simulink model "sim20_8_3"  (R2017a)
settings: Solver=ode45  StartTime=0.0  StopTime=15  FixedStep=0.05  MaxStep=0.05  RelTol=1e-3
libraries: simulink x2
settings Model: Creator=asus  LastModifiedBy=Lenovo

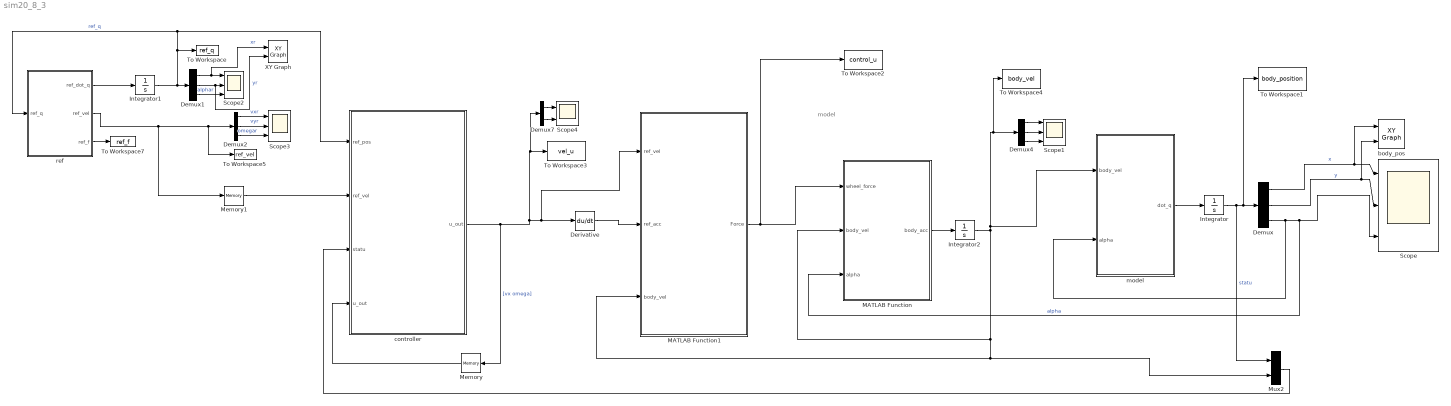
== system sim20_8_3 ==
  note: model
  Demux{,1..2,4} (4 alike) : Demux  Outputs=3
  Demux7 : Demux  Outputs=2
  Derivative : Derivative
  Integrator : Integrator  InitialCondition=[1; -1; pi/2;]  IgnoreLimit=on
  Integrator1 : Integrator  InitialCondition=[0;0;pi/4]
  Integrator2 : Integrator  InitialCondition=[0.2; 0; 0]
  MATLAB Function : MATLAB Function  TreatAsAtomicUnit=on
  MATLAB Function1 : MATLAB Function  TreatAsAtomicUnit=on
  Memory : Memory  X0=[0; 0]
  Memory1 : Memory  X0=[0.00001; 0.00001 ; 0.000001]
  Mux2 : Mux  Inputs=2
  Scope{,1..3} (4 alike) : Scope  NumInputPorts=3
  Scope4 : Scope  NumInputPorts=2
  To Workspace : ToWorkspace  VariableName=ref_q  SampleTime=-1
  To Workspace1 : ToWorkspace  VariableName=body_position  SampleTime=-1
  To Workspace2 : ToWorkspace  VariableName=control_u  SampleTime=-1
  To Workspace3 : ToWorkspace  VariableName=vel_u  SampleTime=-1
  To Workspace4 : ToWorkspace  VariableName=body_vel  SampleTime=-1
  To Workspace5 : ToWorkspace  VariableName=ref_vel  SampleTime=-1
  To Workspace7 : ToWorkspace  VariableName=ref_f  SampleTime=-1
  XY Graph : simulink/Sinks/XY Graph  xmin=-10  xmax=10  ymin=-10  ymax=10  st=-1
  body_pos : simulink/Sinks/XY Graph  xmin=-10  xmax=10  ymin=-10  ymax=10  st=-1
  controller : MATLAB Function  TreatAsAtomicUnit=on
  model : MATLAB Function  TreatAsAtomicUnit=on
  ref : MATLAB Function  TreatAsAtomicUnit=on
  wires:
  Demux2/2 -> Scope3/2  "vyr"
  Demux2/1 -> Scope3/1  "vxr"
  ref/2(ref_vel) -> Memory1/1, To Workspace5/1, Demux2/1
  Integrator/1 -> To Workspace1/1, Demux/1, Mux2/1  "statu"
  Demux1/3 -> Scope2/3  "alphar"
  Demux1/1 -> XY Graph/1, Scope2/1  "xr"
  Demux1/2 -> XY Graph/2, Scope2/2  "yr"
  Demux2/3 -> Scope3/3  "omegar"
  Demux/3 -> model/2(alpha), MATLAB Function/3(alpha), Scope/3  "alpha"
  Demux/1 -> body_pos/1, Scope/1  "x"
  Demux/2 -> body_pos/2, Scope/2  "y"
  ref/1(ref_dot_q) -> Integrator1/1
  Integrator1/1 -> ref/1(ref_q), controller/1(ref_pos), To Workspace/1, Demux1/1  "ref_q"
  Demux7/2 -> Scope4/2
  Demux7/1 -> Scope4/1
  model/1(dot_q) -> Integrator/1
  controller/1(u_out) -> MATLAB Function1/1(ref_vel), Derivative/1, Demux7/1, To Workspace3/1, Memory/1  "[vx omega]"
  Memory/1 -> controller/4("u_out ")
  Memory1/1 -> controller/2(ref_vel)
  ref/3(ref_f) -> To Workspace7/1
  Mux2/1 -> controller/3(statu)
  Integrator2/1 -> Mux2/2, MATLAB Function1/3(body_vel), MATLAB Function/2(body_vel), model/1(body_vel), To Workspace4/1, Demux4/1
  MATLAB Function/1(body_acc) -> Integrator2/1
  Demux4/1 -> Scope1/1
  Demux4/3 -> Scope1/3
  MATLAB Function1/1(Force) -> To Workspace2/1, MATLAB Function/1(wheel_force)
  Demux4/2 -> Scope1/2
  Derivative/1 -> MATLAB Function1/2(ref_acc)

== matlab function sim20_8_3/controller ==
  data: ref_pos input; ref_vel input; u_out output; statu input; u_out input
function u_out  = my_MPC_controller(ref_pos, ref_vel, statu, u_out)

% 程序上没有问题，在运动学模型上是可以完成任务的
% 最近修改时间：7.25 
% 基于运动学模型的MPC控制器
% u_out=[vx ;  omega]
% ref_vel=[xr yr alphar vr omegar]
% e = [ex ey ealpha]

Nc= 10; Np=20; %预测时域Np	控制时域Nc
T=0.05; 

% 测试是否能得到
%    statu=[2; -2; pi/2; 0.001; 0.001; 0.001];
%    u_out=[0; 0];
%    ref_pos=[0;0;pi/4]; ref_vel=[2; 0; 0];  
%% 底盘参数
d = 0.18;	l = 0.16;	m = 24;	Iz = 11.89;	c = 513.6; %轮胎侧偏刚度

%% 状态量                                                                           
x = statu(1);   y = statu(2);  alpha = statu(3); 
vx = statu(4);  vy = statu(5);    omega = statu(6);
                                      
                                                                            
xr=ref_pos(1);  yr=ref_pos(2);  alphar=ref_pos(3);
vxr=ref_vel(1); vyr=ref_vel(2); omegar=ref_vel(3);
                                                                                      
%控制量个数Nu
Nu=size(u_out,1);

%状态量个数Nx
statu_error=[x-xr;   y-yr;   alpha-alphar;]; 
Nx=size(statu_error,1);

% 控制矩阵求解(将连续矩阵转换为离散矩阵，采用近似算法  A=I+T*A(t),B=T*B(t))
% 此处：delta_X=AX+BU ————X=[a-r]=[X_I-Xr;Y_I-Yr;ALPHA_I-ALPHAr]statu_e=A*statu_e+B*u_e   %离散后的模型
    % OUT=delta_X=a-r
A=[ 1 0 -vx*sin(alphar)*T; 0 1 vx*cos(alphar)*T; 0 0 1];
B=[cos(alphar)*T 0 ; sin(alphar)*T 0 ; 0 T];

C = eye(Nx);

Error = C * statu_error; % 误差

% e_pos=Error(1:Nx/2); %位置误差

% 得到新的X=A_new*X+B_new*delta_u   X=[X;u-ur]
A_new = [A B;zeros(Nu,Nx) eye(Nu)];
B_new = [B;eye(Nu)];
C_new = [C,zeros(Nx,Nu)];
%% 
ur=[vxr; omegar];

statu_new = [Error;u_out-ur];

PHI=zeros(Np*size(C_new*A_new,1),size(A_new,2));
for i=1:1:Np
    PHI( Nx*i-(Nx-1):Nx*i  ,:)=C_new*A_new^i;
end

THETA=zeros( Np*size(C_new*B_new,1),  Nc*size(C_new*A_new*B_new ,2) );
for i=1:1:Np
    for j=1:1:Nc
        if j<= i
            THETA( Nx*(i-1)+1:Nx*i,Nu*j-1:Nu*j )= C_new*A_new^(i-j)*B_new;
        else
            THETA( Nx*(i-1)+1:Nx*i,Nu*j-1:Nu*j ) = zeros( Nx,Nu );
        end
    end
end


q = [1 0 0;
     0 1 0;
     0 0 1;];
Q=zeros(Nx*Np,Nx*Np);
for i=1:Np
    for j=1:Np
        if i==j
            Q(Nx*(i-1)+1:Nx*i , Nx*(i-1)+1:Nx*i) = q;
        end
    end
end

R = 1*eye( Nc*Nu,Nc*Nu);

%% 二次型
p=5;

H = [2*THETA'*Q*THETA+R zeros(Nc*Nu,1);zeros(1,Nc*Nu) p];  %不是对称的 % 前面加了个2

ERROR =PHI*statu_new;  
G = [2*ERROR'*Q*THETA zeros(1)];
P_T = ERROR'*Q*ERROR;

%% 约束条件
%控制量约束
M=tril(ones(Nc));
Im= eye(Nu);
A=kron(M,Im); % U=A*DELTA_U+Ut  中的A

Ut=kron(ones(Nc,1),u_out); %Ut

umin=[-5;-2];  %维数与控制变量的个数相同
umax=[ 5; 2];
Umin=kron(ones(Nc,1),umin);
Umax=kron(ones(Nc,1),umax);
a = [A zeros(Nu*Nc,1);-A zeros(Nu*Nc,1)];
b = [Umax-Ut;-Umin+Ut];

 % 状态增量约束
delta_u_range=2;
delta_Umin = kron((-delta_u_range)*ones(Nu,1),ones(Nc,1)); %速度增量约束
delta_Umax = kron( (delta_u_range)*ones(Nu,1),ones(Nc,1));

lb=[delta_Umin;-10];%（求解方程）状态量下界，包含控制时域内控制增量和松弛因子
ub=[delta_Umax;10];%（求解方程）状态量上界，包含控制时域内控制增量和松弛因子
  
%%
coder.extrinsic('quadprog');
coder.extrinsic('tic');
coder.extrinsic('toc');
tic 
[DELTA_U,fval]=quadprog(H,G,a,b,[],[],lb,ub);
toc
% DELTA_U=quadprog(H,G,[],[],[],[],lb,ub)
delta_u = zeros(Nu*Nc+1,1);	% 定义类型，存储DELTA_U的mxarray类型数据
delta_u = DELTA_U;
delta_uout = delta_u(1:2)
u_out = delta_uout+u_out

== matlab function sim20_8_3/model ==
  data: body_vel input; alpha input; dot_q output
function dot_q  = model(body_vel,alpha)


wheel_radius = 0.330/2;
d = 0.18;
l = 0.16;

R = [cos(alpha) -sin(alpha) 0;
     sin(alpha) cos(alpha) 0;
     0 0 1];
% R_w2v =(wheel_radius).*[1/2     1/2;
%                             0           0;
%                         -1/(2*d)  1/(2*d)];
%                     
% max=1/wheel_radius;
% for i=1:size(wheel_omega,2)
%     if wheel_omega(i)>max
%         wheel_omega(i) = max;
%     else
%         if wheel_omega(i)<-max
%             wheel_omega(i) = -max;
%         else
%             wheel_omega(i) = wheel_omega(i);
%         end
%     end
% end
%  wheel_omega;
                    
                    
                    
% body_vel=R_w2v*wheel_omega; % 本体坐标系下的速度

dot_q = R *body_vel; % 世界坐标系下的速度


% 
% 
% x = statu(1);
% y = statu(2);
% alpha = statu(3);
% 
% dot_x = vx*cos(alpha);
% dot_y = vx*sin(alpha);
% dot_alpha = omega;
% 
% 
% 
% % 状态【x y alpha vx vy omega】
% dot_statu = [dot_x; dot_y; dot_alpha];
% vy=0;
% body_vel=[vx;vy; omega]
% 
% 
% end
% 
% % max=1/wheel_radius;
% % for i=1:size(wheel_omega,2)
% %     if wheel_omega(i)>max
% %         wheel_omega(i) = max;
% %     else
% %         if wheel_omega(i)<-max
% %             wheel_omega(i) = -max;
% %         else
% %             wheel_omega(i) = wheel_omega(i);
% %         end
% %     end
% % end

== matlab function sim20_8_3/MATLAB Function ==
  data: wheel_force input; body_acc output; body_vel input; alpha input
function body_acc = dynamic_model(wheel_force,body_vel,alpha)

gravity=[0 0 9.81];

%车辆参数
d = 0.18;
l = 0.16;

m = 24;
Iz = 11.89;

c_wheel = 513.6 ; %侧偏刚度

FX1 = wheel_force(1);    % 将得到的车轮挂钩牵引力分配
FX2 = wheel_force(2);

vx=body_vel(1);
vy=body_vel(2);
omega=body_vel(3);

% beta1=atan( ( vy+l*omega )/( vx+0.000000000000001 ));
% beta2=atan( ( vy+l*omega )/( vx+0.000000000000001 ));

beta1=atan( ( vy+l*omega )/( vx ));
beta2=atan( ( vy+l*omega )/( vx ));

FY1=-c_wheel*beta1;
FY2=-c_wheel*beta2;

dot_vx = ( FX1+FX2 )/m + vy*omega;
dot_vy = ( FY1+FY2 )/m - vx*omega;
dot_omega = ( d*(FX2-FX1)- l*(FY1+FY2) )/Iz;

body_acc=[dot_vx ; dot_vy ; dot_omega]; %得到车辆的加速度

end

== matlab function sim20_8_3/ref ==
  data: ref_q input; ref_dot_q output; ref_vel output; ref_f output
%参考轨迹
%更改时，只需更改vx和Omega即可，实现圆形和直线的不同变化



function [ref_dot_q,ref_vel,ref_f] = fcn(ref_q)
xr=ref_q(1);
yr=ref_q(2);
alphar=ref_q(3);

vxr=1;
vyr=0;
omegar=0.5;

ref_vel=[vxr;vyr;omegar];

dotx = vxr*cos(alphar) - vyr*sin(alphar);
doty = vxr*sin(alphar) + vyr*sin(alphar);
dotalpha = omegar;
ref_dot_q=[dotx;doty;dotalpha];

ref_f = [0;0]
end

== matlab function sim20_8_3/MATLAB Function1 ==
  data: ref_vel input; ref_acc input; Force output; body_vel input
function Force = smc_control(ref_vel,ref_acc,body_vel)
m=24  ;   Iz=11.89     ; d=0.16    ; l=0.18    ;
c_wheel = 513.6 ; %侧偏刚度
vx=body_vel(1);     vy=body_vel(2);     omega=body_vel(3);

%% 参数
C=[1 0; 0 1];
kesi=[0.3 0 ;0 0.3];   K=[0.5 0;0 0.5];

%% 
M=[m 0; 0 Iz];
V=[-m*omega*vy;
    0];

B=[1 1;-d d];
B_=inv(B);

A=[0 -l];

beta1=atan( ( vy+l*omega )/( vx ));
beta2=atan( ( vy+l*omega )/( vx ));

FY1=-c_wheel*beta1;
FY2=-c_wheel*beta2;
body_vel=[body_vel(1); body_vel(2)];
lambda=FY1+FY2;
e=body_vel-ref_vel;
S=C*e;





% slaw = -kesi*sign(S);     %等速趋近律 kesi>0
slaw = -kesi*sign(S)-K*S;   %指数趋近律 kesi>0   k>0
% slaw = -K*abs(S)^a*sign(S); %幂次趋近律 K>0  1>a>0

%将符号函数改为连续函数
delta=0.75;
sfun=S./(abs(S)+delta);

% slaw = -kesi*sfun;     %等速趋近律 kesi>0
slaw = -kesi*sfun-K*S;   %指数趋近律 kesi>0   k>0  为了保证快速趋近的同事削弱抖振，应该增大k的同时减小kesi
% slaw = -K*abs(S)^a*sfun; %幂次趋近律 K>0  1>a>0



u=B_*M*C^(-1)*slaw+B_*V+B_*A'*lambda+B_*M*ref_acc;


Force = u;
